simulink model "ALL_JP360_DBW_V6_5_1103"  (R2022a)
settings: Solver=FixedStepAuto  StartTime=0.0  StopTime=inf  FixedStep=0.01  RelTol=1e-3  EnableMultiTasking=on
model workspace (MAT data in the model file):
  g = 9.8
undefined symbols (not defined in the file or in its folder): canChannel, delta_v_p, IPM_Line_C0, IPM_Line_C1, IPM_Line_C2, IPM_Line_C3, M, M_p, MRR_ObjDistX, MRR_ObjDistY, MRR_ObjFusionCamID, MRR_ObjFusionSig, MRR_ObjID, MRR_ObjRelVelX, MRR_ObjRelVelY, MRR_ObjType, MRR_ObjUpdFlg, none, obj_vaild, untracktime, V, videoinput
libraries: canfdmsglib x230, canfdlib x76, slpidlib x24, simulink x18, dspstat3 x14, ctrlSharedLib x1, simulink_extras x1, imaqlib x1, realtime_pacer_lib x1, dspvision x1, visionsinks x1
(part 53 of 55)

== system ALL_JP360_DBW_V6_5_1103/ACC_Control/ACC_FUNCTION/Subsystem2/Limit/acceleration_throttle——PID/Out_PID/Subsystem11 ==
  acce : Inport
  Action Port : ActionPort  InitializeStates=reset  PropagateVarSize=During execution
  Constant : Constant  Value=100
  Constant1 : Constant  OutDataTypeStr=single
  Constant2 : Constant  OutDataTypeStr=uint8
  Constant4 : Constant  OutDataTypeStr=uint8
  P1 : Gain  Gain=0.08
  P3 : Gain  Gain=0.12
  P4 : Gain  Gain=130
  PID Controller : slpidlib/PID Controller  Controller=PID  Form=Parallel  TimeDomain=Continuous-time  UseExternalTs=off  SampleTime=-1  IntegratorMethod=Forward Euler  FilterMethod=Forward Euler  ControllerParametersSource=external  P=1  I=1  UseKiTs=off  D=0  N=100  UseFilter=on  TunerSelectOption=Transfer Function Based (PID Tuner App)  InitialConditionSource=internal  InitialConditionForIntegrator=0  InitialConditionForFilter=0  DifferentiatorICPrevScaledInput=0  ExternalReset=none  TrackingMode=off  Kt=1  LimitOutput=off  SatLimitsSource=internal  UpperSaturationLimit=inf  LowerSaturationLimit=-inf  LinearizeAsGain=on  AntiWindupMode=none  Kb=1  POutMin=[]  POutMax=[]  IOutMin=[]  IOutMax=[]  DOutMin=[]  DOutMax=[]  NOutMin=[]  NOutMax=[]  SumOutDataTypeStr=single  SumOutMin=[]  SumOutMax=[]  SaturationOutMin=[]  SaturationOutMax=[]  PParamMin=[]  PParamMax=[]  IParamMin=[]  IParamMax=[]  DParamMin=[]  DParamMax=[]  NParamMin=[]  NParamMax=[]  KbParamMin=[]  KbParamMax=[]  KtParamMin=[]  KtParamMax=[]  KbOutMin=[]  KbOutMax=[]  KtOutMin=[]  KtOutMax=[]  IntegratorOutMin=[]  IntegratorOutMax=[]  FilterOutMin=[]  FilterOutMax=[]  SumI1OutMin=[]  SumI1OutMax=[]  SumI2OutMin=[]  SumI2OutMax=[]  SumI3OutMin=[]  SumI3OutMax=[]  SumI4OutMin=[]  SumI4OutMax=[]  SumDOutMin=[]  SumDOutMax=[]  DifferentiatorOutMin=[]  DifferentiatorOutMax=[]  FilterDiffOutCoefMin=[]  FilterDiffOutCoefMax=[]  ReciprocalOutMin=[]  ReciprocalOutMax=[]  SumDenOutMin=[]  SumDenOutMax=[]  SumNumOutMin=[]  SumNumOutMax=[]  DivideOutMin=[]  DivideOutMax=[]  UdiffTsProdOutMin=[]  UdiffTsProdOutMax=[]  NTsProdOutMin=[]  NTsProdOutMax=[]  UintegralTsProdOutMin=[]  UintegralTsProdOutMax=[]  UngainTsProdOutMin=[]  UngainTsProdOutMax=[]  IntegratorContinuousStateAttributes=''  IntegratorStateMustResolveToSignalObject=off  IntegratorRTWStateStorageClass=Auto  FilterContinuousStateAttributes=''  FilterStateMustResolveToSignalObject=off  FilterRTWStateStorageClass=Auto  ParallelPVariant=ExternalParameters  IdealPVariant=Disabled  IVariant=ExternalParameters  DVariant=ExternalParameters  IntegratorVariant=Continuous  SatVariant=Disabled  AWVariant=Passthrough  PCopyVariant=Disabled  TRVariant=Disabled  FdbkBlocksVariant=Forward  IdealPFdbkVariant=Disabled  SatFdbkVariant=Disabled  DerivativeFilterVariant=ContFilter  NVariant=ExternalParameters  NCopyVariant=Disabled  FilterICVariant=InternalICsFilter  IntegratorICVariant=InternalICs  ExternalResetVariant=Disabled  TRSumVariant=Passthrough  SumFdbkVariant=Disabled  SumVariant=Sum_PID  TsampFilterVariant=InternalTs  TsampNgainVariant=Passthrough  TsampIntegralVariant=Passthrough  ExternalSaturationOutDataTypeStr=Inherit: Same as second input  aMode=0
  Out1 : Outport
  wires:
  PID Controller/1 -> Out1/1  "throttle"
  acce/1 -> PID Controller/1  "err_v"
  P3/1 -> PID Controller/3
  Constant/1 -> PID Controller/5
  Constant4/1 -> P4/1
  Constant2/1 -> P1/1
  Constant1/1 -> P3/1
  P1/1 -> PID Controller/4
  P4/1 -> PID Controller/2

== system ALL_JP360_DBW_V6_5_1103/ACC_Control/ACC_FUNCTION/Subsystem2/Limit/acceleration_throttle——PID/Out_PID/Subsystem12 ==
  acce : Inport
  Action Port : ActionPort  InitializeStates=reset  PropagateVarSize=During execution
  Constant : Constant  Value=100
  Constant1 : Constant  OutDataTypeStr=single
  Constant2 : Constant  OutDataTypeStr=uint8
  Constant4 : Constant  OutDataTypeStr=uint8
  P1 : Gain  Gain=0.08
  P3 : Gain  Gain=0.12
  P4 : Gain  Gain=130
  PID Controller : slpidlib/PID Controller  Controller=PID  Form=Parallel  TimeDomain=Continuous-time  UseExternalTs=off  SampleTime=-1  IntegratorMethod=Forward Euler  FilterMethod=Forward Euler  ControllerParametersSource=external  P=1  I=1  UseKiTs=off  D=0  N=100  UseFilter=on  TunerSelectOption=Transfer Function Based (PID Tuner App)  InitialConditionSource=internal  InitialConditionForIntegrator=0  InitialConditionForFilter=0  DifferentiatorICPrevScaledInput=0  ExternalReset=none  TrackingMode=off  Kt=1  LimitOutput=off  SatLimitsSource=internal  UpperSaturationLimit=inf  LowerSaturationLimit=-inf  LinearizeAsGain=on  AntiWindupMode=none  Kb=1  POutMin=[]  POutMax=[]  IOutMin=[]  IOutMax=[]  DOutMin=[]  DOutMax=[]  NOutMin=[]  NOutMax=[]  SumOutDataTypeStr=single  SumOutMin=[]  SumOutMax=[]  SaturationOutMin=[]  SaturationOutMax=[]  PParamMin=[]  PParamMax=[]  IParamMin=[]  IParamMax=[]  DParamMin=[]  DParamMax=[]  NParamMin=[]  NParamMax=[]  KbParamMin=[]  KbParamMax=[]  KtParamMin=[]  KtParamMax=[]  KbOutMin=[]  KbOutMax=[]  KtOutMin=[]  KtOutMax=[]  IntegratorOutMin=[]  IntegratorOutMax=[]  FilterOutMin=[]  FilterOutMax=[]  SumI1OutMin=[]  SumI1OutMax=[]  SumI2OutMin=[]  SumI2OutMax=[]  SumI3OutMin=[]  SumI3OutMax=[]  SumI4OutMin=[]  SumI4OutMax=[]  SumDOutMin=[]  SumDOutMax=[]  DifferentiatorOutMin=[]  DifferentiatorOutMax=[]  FilterDiffOutCoefMin=[]  FilterDiffOutCoefMax=[]  ReciprocalOutMin=[]  ReciprocalOutMax=[]  SumDenOutMin=[]  SumDenOutMax=[]  SumNumOutMin=[]  SumNumOutMax=[]  DivideOutMin=[]  DivideOutMax=[]  UdiffTsProdOutMin=[]  UdiffTsProdOutMax=[]  NTsProdOutMin=[]  NTsProdOutMax=[]  UintegralTsProdOutMin=[]  UintegralTsProdOutMax=[]  UngainTsProdOutMin=[]  UngainTsProdOutMax=[]  IntegratorContinuousStateAttributes=''  IntegratorStateMustResolveToSignalObject=off  IntegratorRTWStateStorageClass=Auto  FilterContinuousStateAttributes=''  FilterStateMustResolveToSignalObject=off  FilterRTWStateStorageClass=Auto  ParallelPVariant=ExternalParameters  IdealPVariant=Disabled  IVariant=ExternalParameters  DVariant=ExternalParameters  IntegratorVariant=Continuous  SatVariant=Disabled  AWVariant=Passthrough  PCopyVariant=Disabled  TRVariant=Disabled  FdbkBlocksVariant=Forward  IdealPFdbkVariant=Disabled  SatFdbkVariant=Disabled  DerivativeFilterVariant=ContFilter  NVariant=ExternalParameters  NCopyVariant=Disabled  FilterICVariant=InternalICsFilter  IntegratorICVariant=InternalICs  ExternalResetVariant=Disabled  TRSumVariant=Passthrough  SumFdbkVariant=Disabled  SumVariant=Sum_PID  TsampFilterVariant=InternalTs  TsampNgainVariant=Passthrough  TsampIntegralVariant=Passthrough  ExternalSaturationOutDataTypeStr=Inherit: Same as second input  aMode=0
  Out1 : Outport
  wires:
  P4/1 -> PID Controller/2
  P1/1 -> PID Controller/4
  Constant1/1 -> P3/1
  Constant2/1 -> P1/1
  Constant4/1 -> P4/1
  Constant/1 -> PID Controller/5
  P3/1 -> PID Controller/3
  acce/1 -> PID Controller/1  "err_v"
  PID Controller/1 -> Out1/1  "throttle"

== system ALL_JP360_DBW_V6_5_1103/ACC_Control/ACC_FUNCTION/Subsystem2/Limit/acceleration_throttle——PID/Out_PID/Subsystem13 ==
  Action Port : ActionPort  InitializeStates=reset  PropagateVarSize=During execution
  Constant3 : Constant  Value=25  OutDataTypeStr=uint8
  Data Type Conversion : DataTypeConversion  OutDataTypeStr=single  SaturateOnIntegerOverflow=off  RndMeth=Floor
  Out1 : Outport
  wires:
  Data Type Conversion/1 -> Out1/1
  Constant3/1 -> Data Type Conversion/1  "throttle"

== system ALL_JP360_DBW_V6_5_1103/ACC_Control/ACC_FUNCTION/Subsystem2/Limit/acceleration_throttle——PID/Out_PID/Subsystem2 ==
  Action Port : ActionPort  InitializeStates=reset  PropagateVarSize=During execution
  Constant1 : Constant  Value=0  OutDataTypeStr=single
  Constant3 : Constant  Value=25  OutDataTypeStr=uint8
  Data Type Conversion : DataTypeConversion  OutDataTypeStr=single  SaturateOnIntegerOverflow=off  RndMeth=Floor
  Out1 : Outport
  Out2 : Outport  Port=2
  wires:
  Constant1/1 -> Out2/1  "throttle"
  Constant3/1 -> Data Type Conversion/1  "throttle"
  Data Type Conversion/1 -> Out1/1

== system ALL_JP360_DBW_V6_5_1103/ACC_Control/ACC_FUNCTION/Subsystem2/Limit/acceleration_throttle——PID/Out_PID/up81 ==
  acce : Inport
  Action Port : ActionPort  InitializeStates=reset  PropagateVarSize=During execution
  Constant : Constant  Value=100  OutDataTypeStr=int8
  Constant1 : Constant  OutDataTypeStr=uint16
  Constant2 : Constant  OutDataTypeStr=uint16
  Constant3 : Constant  Value=81  OutDataTypeStr=single
  Constant4 : Constant  OutDataTypeStr=uint8
  P1 : Gain  Gain=0
  P3 : Gain  Gain=6
  P4 : Gain  Gain=145
  PID Controller : slpidlib/PID Controller  Controller=PID  Form=Parallel  TimeDomain=Continuous-time  UseExternalTs=off  SampleTime=-1  IntegratorMethod=Forward Euler  FilterMethod=Forward Euler  ControllerParametersSource=external  P=1  I=1  UseKiTs=off  D=0  N=100  UseFilter=on  TunerSelectOption=Transfer Function Based (PID Tuner App)  InitialConditionSource=internal  InitialConditionForIntegrator=0  InitialConditionForFilter=0  DifferentiatorICPrevScaledInput=0  ExternalReset=none  TrackingMode=off  Kt=1  LimitOutput=off  SatLimitsSource=internal  UpperSaturationLimit=inf  LowerSaturationLimit=-inf  LinearizeAsGain=on  AntiWindupMode=none  Kb=1  POutMin=[]  POutMax=[]  IOutMin=[]  IOutMax=[]  DOutMin=[]  DOutMax=[]  NOutMin=[]  NOutMax=[]  SumOutDataTypeStr=single  SumOutMin=[]  SumOutMax=[]  SaturationOutMin=[]  SaturationOutMax=[]  PParamMin=[]  PParamMax=[]  IParamMin=[]  IParamMax=[]  DParamMin=[]  DParamMax=[]  NParamMin=[]  NParamMax=[]  KbParamMin=[]  KbParamMax=[]  KtParamMin=[]  KtParamMax=[]  KbOutMin=[]  KbOutMax=[]  KtOutMin=[]  KtOutMax=[]  IntegratorOutMin=[]  IntegratorOutMax=[]  FilterOutMin=[]  FilterOutMax=[]  SumI1OutMin=[]  SumI1OutMax=[]  SumI2OutMin=[]  SumI2OutMax=[]  SumI3OutMin=[]  SumI3OutMax=[]  SumI4OutMin=[]  SumI4OutMax=[]  SumDOutMin=[]  SumDOutMax=[]  DifferentiatorOutMin=[]  DifferentiatorOutMax=[]  FilterDiffOutCoefMin=[]  FilterDiffOutCoefMax=[]  ReciprocalOutMin=[]  ReciprocalOutMax=[]  SumDenOutMin=[]  SumDenOutMax=[]  SumNumOutMin=[]  SumNumOutMax=[]  DivideOutMin=[]  DivideOutMax=[]  UdiffTsProdOutMin=[]  UdiffTsProdOutMax=[]  NTsProdOutMin=[]  NTsProdOutMax=[]  UintegralTsProdOutMin=[]  UintegralTsProdOutMax=[]  UngainTsProdOutMin=[]  UngainTsProdOutMax=[]  IntegratorContinuousStateAttributes=''  IntegratorStateMustResolveToSignalObject=off  IntegratorRTWStateStorageClass=Auto  FilterContinuousStateAttributes=''  FilterStateMustResolveToSignalObject=off  FilterRTWStateStorageClass=Auto  ParallelPVariant=ExternalParameters  IdealPVariant=Disabled  IVariant=ExternalParameters  DVariant=ExternalParameters  IntegratorVariant=Continuous  SatVariant=Disabled  AWVariant=Passthrough  PCopyVariant=Disabled  TRVariant=Disabled  FdbkBlocksVariant=Forward  IdealPFdbkVariant=Disabled  SatFdbkVariant=Disabled  DerivativeFilterVariant=ContFilter  NVariant=ExternalParameters  NCopyVariant=Disabled  FilterICVariant=InternalICsFilter  IntegratorICVariant=InternalICs  ExternalResetVariant=Disabled  TRSumVariant=Passthrough  SumFdbkVariant=Disabled  SumVariant=Sum_PID  TsampFilterVariant=InternalTs  TsampNgainVariant=Passthrough  TsampIntegralVariant=Passthrough  ExternalSaturationOutDataTypeStr=Inherit: Same as second input  aMode=0
  Out1 : Outport
  Out2 : Outport  Port=2
  wires:
  Constant3/1 -> Out2/1  "throttle"
  P4/1 -> PID Controller/2
  P1/1 -> PID Controller/4
  Constant1/1 -> P3/1
  Constant2/1 -> P1/1
  Constant4/1 -> P4/1
  Constant/1 -> PID Controller/5
  P3/1 -> PID Controller/3
  acce/1 -> PID Controller/1  "err_v"
  PID Controller/1 -> Out1/1  "throttle"

== system ALL_JP360_DBW_V6_5_1103/ACC_Control/ACC_FUNCTION/Subsystem2/Limit/acceleration_throttle——PID/Subsystem2/30-50 ==
  acce : Inport
  Action Port : ActionPort  InitializeStates=reset  PropagateVarSize=During execution
  Constant : Constant  Value=100
  Constant1 : Constant  OutDataTypeStr=single
  Constant2 : Constant  OutDataTypeStr=uint8
  Constant3 : Constant  Value=100  OutDataTypeStr=single
  Constant4 : Constant  OutDataTypeStr=uint8
  P1 : Gain  Gain=0
  P3 : Gain  Gain=3
  P4 : Gain  Gain=110
  PID Controller : slpidlib/PID Controller  Controller=PID  Form=Parallel  TimeDomain=Continuous-time  UseExternalTs=off  SampleTime=-1  IntegratorMethod=Forward Euler  FilterMethod=Forward Euler  ControllerParametersSource=external  P=1  I=1  UseKiTs=off  D=0  N=100  UseFilter=on  TunerSelectOption=Transfer Function Based (PID Tuner App)  InitialConditionSource=internal  InitialConditionForIntegrator=0  InitialConditionForFilter=0  DifferentiatorICPrevScaledInput=0  ExternalReset=none  TrackingMode=off  Kt=1  LimitOutput=off  SatLimitsSource=internal  UpperSaturationLimit=inf  LowerSaturationLimit=-inf  LinearizeAsGain=on  AntiWindupMode=none  Kb=1  POutMin=[]  POutMax=[]  IOutMin=[]  IOutMax=[]  DOutMin=[]  DOutMax=[]  NOutMin=[]  NOutMax=[]  SumOutDataTypeStr=single  SumOutMin=[]  SumOutMax=[]  SaturationOutMin=[]  SaturationOutMax=[]  PParamMin=[]  PParamMax=[]  IParamMin=[]  IParamMax=[]  DParamMin=[]  DParamMax=[]  NParamMin=[]  NParamMax=[]  KbParamMin=[]  KbParamMax=[]  KtParamMin=[]  KtParamMax=[]  KbOutMin=[]  KbOutMax=[]  KtOutMin=[]  KtOutMax=[]  IntegratorOutMin=[]  IntegratorOutMax=[]  FilterOutMin=[]  FilterOutMax=[]  SumI1OutMin=[]  SumI1OutMax=[]  SumI2OutMin=[]  SumI2OutMax=[]  SumI3OutMin=[]  SumI3OutMax=[]  SumI4OutMin=[]  SumI4OutMax=[]  SumDOutMin=[]  SumDOutMax=[]  DifferentiatorOutMin=[]  DifferentiatorOutMax=[]  FilterDiffOutCoefMin=[]  FilterDiffOutCoefMax=[]  ReciprocalOutMin=[]  ReciprocalOutMax=[]  SumDenOutMin=[]  SumDenOutMax=[]  SumNumOutMin=[]  SumNumOutMax=[]  DivideOutMin=[]  DivideOutMax=[]  UdiffTsProdOutMin=[]  UdiffTsProdOutMax=[]  NTsProdOutMin=[]  NTsProdOutMax=[]  UintegralTsProdOutMin=[]  UintegralTsProdOutMax=[]  UngainTsProdOutMin=[]  UngainTsProdOutMax=[]  IntegratorContinuousStateAttributes=''  IntegratorStateMustResolveToSignalObject=off  IntegratorRTWStateStorageClass=Auto  FilterContinuousStateAttributes=''  FilterStateMustResolveToSignalObject=off  FilterRTWStateStorageClass=Auto  ParallelPVariant=ExternalParameters  IdealPVariant=Disabled  IVariant=ExternalParameters  DVariant=ExternalParameters  IntegratorVariant=Continuous  SatVariant=Disabled  AWVariant=Passthrough  PCopyVariant=Disabled  TRVariant=Disabled  FdbkBlocksVariant=Forward  IdealPFdbkVariant=Disabled  SatFdbkVariant=Disabled  DerivativeFilterVariant=ContFilter  NVariant=ExternalParameters  NCopyVariant=Disabled  FilterICVariant=InternalICsFilter  IntegratorICVariant=InternalICs  ExternalResetVariant=Disabled  TRSumVariant=Passthrough  SumFdbkVariant=Disabled  SumVariant=Sum_PID  TsampFilterVariant=InternalTs  TsampNgainVariant=Passthrough  TsampIntegralVariant=Passthrough  ExternalSaturationOutDataTypeStr=Inherit: Same as second input  aMode=0
  Out1 : Outport
  Out2 : Outport  Port=2
  wires:
  Constant3/1 -> Out2/1
  P4/1 -> PID Controller/2
  P1/1 -> PID Controller/4
  Constant1/1 -> P3/1
  Constant2/1 -> P1/1
  Constant4/1 -> P4/1
  Constant/1 -> PID Controller/5
  P3/1 -> PID Controller/3
  acce/1 -> PID Controller/1  "err_v"
  PID Controller/1 -> Out1/1  "throttle"

== system ALL_JP360_DBW_V6_5_1103/ACC_Control/ACC_FUNCTION/Subsystem2/Limit/acceleration_throttle——PID/Subsystem2/51-80 ==
  acce : Inport
  Action Port : ActionPort  InitializeStates=reset  PropagateVarSize=During execution
  Constant : Constant  Value=100
  Constant1 : Constant  OutDataTypeStr=single
  Constant2 : Constant  OutDataTypeStr=uint8
  Constant3 : Constant  Value=200  OutDataTypeStr=single
  Constant4 : Constant  OutDataTypeStr=uint8
  P1 : Gain  Gain=0
  P3 : Gain  Gain=5
  P4 : Gain  Gain=135
  PID Controller : slpidlib/PID Controller  Controller=PID  Form=Parallel  TimeDomain=Continuous-time  UseExternalTs=off  SampleTime=-1  IntegratorMethod=Forward Euler  FilterMethod=Forward Euler  ControllerParametersSource=external  P=1  I=1  UseKiTs=off  D=0  N=100  UseFilter=on  TunerSelectOption=Transfer Function Based (PID Tuner App)  InitialConditionSource=internal  InitialConditionForIntegrator=0  InitialConditionForFilter=0  DifferentiatorICPrevScaledInput=0  ExternalReset=none  TrackingMode=off  Kt=1  LimitOutput=off  SatLimitsSource=internal  UpperSaturationLimit=inf  LowerSaturationLimit=-inf  LinearizeAsGain=on  AntiWindupMode=none  Kb=1  POutMin=[]  POutMax=[]  IOutMin=[]  IOutMax=[]  DOutMin=[]  DOutMax=[]  NOutMin=[]  NOutMax=[]  SumOutDataTypeStr=single  SumOutMin=[]  SumOutMax=[]  SaturationOutMin=[]  SaturationOutMax=[]  PParamMin=[]  PParamMax=[]  IParamMin=[]  IParamMax=[]  DParamMin=[]  DParamMax=[]  NParamMin=[]  NParamMax=[]  KbParamMin=[]  KbParamMax=[]  KtParamMin=[]  KtParamMax=[]  KbOutMin=[]  KbOutMax=[]  KtOutMin=[]  KtOutMax=[]  IntegratorOutMin=[]  IntegratorOutMax=[]  FilterOutMin=[]  FilterOutMax=[]  SumI1OutMin=[]  SumI1OutMax=[]  SumI2OutMin=[]  SumI2OutMax=[]  SumI3OutMin=[]  SumI3OutMax=[]  SumI4OutMin=[]  SumI4OutMax=[]  SumDOutMin=[]  SumDOutMax=[]  DifferentiatorOutMin=[]  DifferentiatorOutMax=[]  FilterDiffOutCoefMin=[]  FilterDiffOutCoefMax=[]  ReciprocalOutMin=[]  ReciprocalOutMax=[]  SumDenOutMin=[]  SumDenOutMax=[]  SumNumOutMin=[]  SumNumOutMax=[]  DivideOutMin=[]  DivideOutMax=[]  UdiffTsProdOutMin=[]  UdiffTsProdOutMax=[]  NTsProdOutMin=[]  NTsProdOutMax=[]  UintegralTsProdOutMin=[]  UintegralTsProdOutMax=[]  UngainTsProdOutMin=[]  UngainTsProdOutMax=[]  IntegratorContinuousStateAttributes=''  IntegratorStateMustResolveToSignalObject=off  IntegratorRTWStateStorageClass=Auto  FilterContinuousStateAttributes=''  FilterStateMustResolveToSignalObject=off  FilterRTWStateStorageClass=Auto  ParallelPVariant=ExternalParameters  IdealPVariant=Disabled  IVariant=ExternalParameters  DVariant=ExternalParameters  IntegratorVariant=Continuous  SatVariant=Disabled  AWVariant=Passthrough  PCopyVariant=Disabled  TRVariant=Disabled  FdbkBlocksVariant=Forward  IdealPFdbkVariant=Disabled  SatFdbkVariant=Disabled  DerivativeFilterVariant=ContFilter  NVariant=ExternalParameters  NCopyVariant=Disabled  FilterICVariant=InternalICsFilter  IntegratorICVariant=InternalICs  ExternalResetVariant=Disabled  TRSumVariant=Passthrough  SumFdbkVariant=Disabled  SumVariant=Sum_PID  TsampFilterVariant=InternalTs  TsampNgainVariant=Passthrough  TsampIntegralVariant=Passthrough  ExternalSaturationOutDataTypeStr=Inherit: Same as second input  aMode=0
  Out1 : Outport
  Out2 : Outport  Port=2
  wires:
  Constant3/1 -> Out2/1
  PID Controller/1 -> Out1/1  "throttle"
  acce/1 -> PID Controller/1  "err_v"
  P3/1 -> PID Controller/3
  Constant/1 -> PID Controller/5
  Constant4/1 -> P4/1
  Constant2/1 -> P1/1
  Constant1/1 -> P3/1
  P1/1 -> PID Controller/4
  P4/1 -> PID Controller/2

== system ALL_JP360_DBW_V6_5_1103/ACC_Control/ACC_FUNCTION/Subsystem2/Limit/acceleration_throttle——PID/Subsystem2/up81 ==
  acce : Inport
  Action Port : ActionPort  InitializeStates=reset  PropagateVarSize=During execution
  Constant : Constant  Value=100  OutDataTypeStr=int8
  Constant1 : Constant  OutDataTypeStr=uint16
  Constant2 : Constant  OutDataTypeStr=uint16
  Constant3 : Constant  Value=300  OutDataTypeStr=single
  Constant4 : Constant  OutDataTypeStr=uint8
  P1 : Gain  Gain=0
  P3 : Gain  Gain=5.5
  P4 : Gain  Gain=130
  PID Controller : slpidlib/PID Controller  Controller=PID  Form=Parallel  TimeDomain=Continuous-time  UseExternalTs=off  SampleTime=-1  IntegratorMethod=Forward Euler  FilterMethod=Forward Euler  ControllerParametersSource=external  P=1  I=1  UseKiTs=off  D=0  N=100  UseFilter=on  TunerSelectOption=Transfer Function Based (PID Tuner App)  InitialConditionSource=internal  InitialConditionForIntegrator=0  InitialConditionForFilter=0  DifferentiatorICPrevScaledInput=0  ExternalReset=none  TrackingMode=off  Kt=1  LimitOutput=off  SatLimitsSource=internal  UpperSaturationLimit=inf  LowerSaturationLimit=-inf  LinearizeAsGain=on  AntiWindupMode=none  Kb=1  POutMin=[]  POutMax=[]  IOutMin=[]  IOutMax=[]  DOutMin=[]  DOutMax=[]  NOutMin=[]  NOutMax=[]  SumOutDataTypeStr=single  SumOutMin=[]  SumOutMax=[]  SaturationOutMin=[]  SaturationOutMax=[]  PParamMin=[]  PParamMax=[]  IParamMin=[]  IParamMax=[]  DParamMin=[]  DParamMax=[]  NParamMin=[]  NParamMax=[]  KbParamMin=[]  KbParamMax=[]  KtParamMin=[]  KtParamMax=[]  KbOutMin=[]  KbOutMax=[]  KtOutMin=[]  KtOutMax=[]  IntegratorOutMin=[]  IntegratorOutMax=[]  FilterOutMin=[]  FilterOutMax=[]  SumI1OutMin=[]  SumI1OutMax=[]  SumI2OutMin=[]  SumI2OutMax=[]  SumI3OutMin=[]  SumI3OutMax=[]  SumI4OutMin=[]  SumI4OutMax=[]  SumDOutMin=[]  SumDOutMax=[]  DifferentiatorOutMin=[]  DifferentiatorOutMax=[]  FilterDiffOutCoefMin=[]  FilterDiffOutCoefMax=[]  ReciprocalOutMin=[]  ReciprocalOutMax=[]  SumDenOutMin=[]  SumDenOutMax=[]  SumNumOutMin=[]  SumNumOutMax=[]  DivideOutMin=[]  DivideOutMax=[]  UdiffTsProdOutMin=[]  UdiffTsProdOutMax=[]  NTsProdOutMin=[]  NTsProdOutMax=[]  UintegralTsProdOutMin=[]  UintegralTsProdOutMax=[]  UngainTsProdOutMin=[]  UngainTsProdOutMax=[]  IntegratorContinuousStateAttributes=''  IntegratorStateMustResolveToSignalObject=off  IntegratorRTWStateStorageClass=Auto  FilterContinuousStateAttributes=''  FilterStateMustResolveToSignalObject=off  FilterRTWStateStorageClass=Auto  ParallelPVariant=ExternalParameters  IdealPVariant=Disabled  IVariant=ExternalParameters  DVariant=ExternalParameters  IntegratorVariant=Continuous  SatVariant=Disabled  AWVariant=Passthrough  PCopyVariant=Disabled  TRVariant=Disabled  FdbkBlocksVariant=Forward  IdealPFdbkVariant=Disabled  SatFdbkVariant=Disabled  DerivativeFilterVariant=ContFilter  NVariant=ExternalParameters  NCopyVariant=Disabled  FilterICVariant=InternalICsFilter  IntegratorICVariant=InternalICs  ExternalResetVariant=Disabled  TRSumVariant=Passthrough  SumFdbkVariant=Disabled  SumVariant=Sum_PID  TsampFilterVariant=InternalTs  TsampNgainVariant=Passthrough  TsampIntegralVariant=Passthrough  ExternalSaturationOutDataTypeStr=Inherit: Same as second input  aMode=0
  Out1 : Outport
  Out2 : Outport  Port=2
  wires:
  Constant3/1 -> Out2/1
  P4/1 -> PID Controller/2
  P1/1 -> PID Controller/4
  Constant1/1 -> P3/1
  Constant2/1 -> P1/1
  Constant4/1 -> P4/1
  Constant/1 -> PID Controller/5
  P3/1 -> PID Controller/3
  acce/1 -> PID Controller/1  "err_v"
  PID Controller/1 -> Out1/1  "throttle"

== system ALL_JP360_DBW_V6_5_1103/ACC_Control/ACC_FUNCTION/Subsystem2/ACC_model/TIS1 ACC action/Subsystem1/mode change/cc ==
  throttle_in : Inport
  brake_in : Inport  Port=2
  Action Port : ActionPort  InitializeStates=reset  PropagateVarSize=During execution  ActionPortLabel=if(u1 > 0)
  Constant : Constant  Value=2  OutDataTypeStr=single
  acceleration [a] : Outport  InitialOutput=[0]
  deceleration [-a] : Outport  Port=2  InitialOutput=[150]
  ACC_MODE : Outport  Port=3  InitialOutput=[150]
  wires:
  brake_in/1 -> deceleration [-a]/1
  throttle_in/1 -> acceleration [a]/1
  Constant/1 -> ACC_MODE/1

== system ALL_JP360_DBW_V6_5_1103/ACC_Control/ACC_FUNCTION/Subsystem2/ACC_model/TIS1 ACC action/Subsystem1/mode change/cc and close and follow ==
  a_zero : Inport
  v_obj : Inport  Port=2
  v_ego : Inport  Port=3
  cc_throttle : Inport  Port=4
  cc_brake : Inport  Port=5
  delta_d_ego : Inport  Port=6
  dx : Inport  Port=7
  Action Port : ActionPort  InitializeStates=reset  PropagateVarSize=During execution  ActionPortLabel=else
  Demux : Demux  Outputs=3
  Merge : Merge
  Mux : Mux  Inputs=3
  Mux2 : Mux  Inputs=3
  cc and close : Subsystem  TreatAsAtomicUnit=on
  follow : Subsystem  TreatAsAtomicUnit=on
  if : If
  acceleration [a] : Outport
  deceleration [-a] : Outport  Port=2
  ACC_MODE : Outport  Port=3
  standstill_req : Outport  Port=4  InitialOutput=[150]
  wires:
  follow/1(acceleration [a]) -> Mux2/1
  if/1 -> cc and close/Action
  Demux/1 -> acceleration [a]/1
  cc and close/2(deceleration [-a]) -> Mux/2
  follow/2(deceleration [-a]) -> Mux2/2
  cc and close/1(acceleration [a]) -> Mux/1
  Merge/1 -> Demux/1
  if/2 -> follow/Action
  Mux/1 -> Merge/1
  Demux/2 -> deceleration [-a]/1
  Mux2/1 -> Merge/2
  v_obj/1 -> cc and close/1(v_obj)
  v_ego/1 -> cc and close/2(v_ego)
  a_zero/1 -> follow/1(brake), if/1
  cc_throttle/1 -> cc and close/3(cc_throttle)
  cc_brake/1 -> cc and close/4(cc_brake)
  delta_d_ego/1 -> cc and close/5(delta_d_ego)
  follow/3(ACC_MODE) -> Mux2/3
  cc and close/3(ACC_MODE) -> Mux/3
  Demux/3 -> ACC_MODE/1
  cc and close/4(standstill_req) -> standstill_req/1
  dx/1 -> cc and close/6(dx)

== system ALL_JP360_DBW_V6_5_1103/ACC_Control/ACC_FUNCTION/Subsystem2/ACC_model/TIS1 ACC action/Subsystem1/mode change/cc and close and follow/cc and close ==
  v_obj : Inport
  v_ego : Inport  Port=2
  cc_throttle : Inport  Port=3
  cc_brake : Inport  Port=4
  delta_d_ego : Inport  Port=5
  dx : Inport  Port=6
  Action Port : ActionPort  InitializeStates=reset  PropagateVarSize=During execution  ActionPortLabel=if(u1 > 0)
  Demux : Demux  Outputs=3
  Merge : Merge
  Mux : Mux  Inputs=3
  Mux2 : Mux  Inputs=3
  Sum : Sum  Inputs=|+-
  cc : Subsystem  TreatAsAtomicUnit=on
  if : If
  move close : Subsystem  TreatAsAtomicUnit=on
  acceleration [a] : Outport  OutDataTypeStr=single  InitialOutput=[0]
  deceleration [-a] : Outport  Port=2  OutDataTypeStr=single  InitialOutput=[150]
  ACC_MODE : Outport  Port=3  OutDataTypeStr=single  InitialOutput=[150]
  standstill_req : Outport  Port=4  InitialOutput=[150]
  wires:
  move close/1(acceleration [a]) -> Mux2/1
  Mux2/1 -> Merge/2
  Mux/1 -> Merge/1
  Merge/1 -> Demux/1
  cc/2(deceleration [-a]) -> Mux/2
  if/2 -> move close/Action
  if/1 -> cc/Action
  move close/2(decleration [-a]) -> Mux2/2
  Demux/2 -> deceleration [-a]/1
  Demux/1 -> acceleration [a]/1
  v_obj/1 -> move close/3(v_obj), Sum/1
  v_ego/1 -> move close/4(v_ego), Sum/2
  Sum/1 -> move close/2(delta_v), if/1
  cc_throttle/1 -> cc/1(cc_throttle), move close/5(cc_throttle)
  cc_brake/1 -> move close/6(cc_brake), cc/2(cc_brake)
  delta_d_ego/1 -> move close/1(delta_d_ego)
  cc/3(ACC_MODE) -> Mux/3
  move close/3(ACC_MODE) -> Mux2/3
  Demux/3 -> ACC_MODE/1
  cc/1(acceleration [a]) -> Mux/1
  move close/4(standstill_req) -> standstill_req/1
  dx/1 -> move close/7(dx)

== system ALL_JP360_DBW_V6_5_1103/ACC_Control/ACC_FUNCTION/Subsystem2/ACC_model/TIS1 ACC action/Subsystem1/mode change/cc and close and follow/follow ==
  brake : Inport
  Action Port : ActionPort  InitializeStates=reset  PropagateVarSize=During execution  ActionPortLabel=else
  Constant : Constant  Value=0  OutDataTypeStr=single
  Constant1 : Constant  Value=4  OutDataTypeStr=single
  Saturation : Saturate  UpperLimit=0  LowerLimit=-8
  acceleration [a] : Outport  InitialOutput=[0]
  deceleration [-a] : Outport  Port=2  InitialOutput=[150]
  ACC_MODE : Outport  Port=3  InitialOutput=[0]
  wires:
  Constant/1 -> acceleration [a]/1
  brake/1 -> Saturation/1
  Constant1/1 -> ACC_MODE/1
  Saturation/1 -> deceleration [-a]/1

== system ALL_JP360_DBW_V6_5_1103/ACC_Control/ACC_FUNCTION/Subsystem2/ACC_model/TIS1 ACC action/Subsystem1/mode change/cc and close and follow/cc and close/cc ==
  cc_throttle : Inport
  cc_brake : Inport  Port=2
  Action Port : ActionPort  InitializeStates=reset  PropagateVarSize=During execution  ActionPortLabel=if(u1 > 0)
  Constant : Constant  Value=2  OutDataTypeStr=single
  acceleration [a] : Outport  InitialOutput=[0]
  deceleration [-a] : Outport  Port=2  InitialOutput=[150]
  ACC_MODE : Outport  Port=3  InitialOutput=[150]
  wires:
  cc_throttle/1 -> acceleration [a]/1
  cc_brake/1 -> deceleration [-a]/1
  Constant/1 -> ACC_MODE/1

== system ALL_JP360_DBW_V6_5_1103/ACC_Control/ACC_FUNCTION/Subsystem2/ACC_model/TIS1 ACC action/Subsystem1/mode change/cc and close and follow/cc and close/move close ==
  note: 跟停前车时，若在跟进模式下，目标车静止<10kph，且自车车速＜2kph，发出standstill请求
  delta_d_ego : Inport
  delta_v : Inport  Port=2
  v_obj : Inport  Port=3
  v_ego : Inport  Port=4
  cc_throttle : Inport  Port=5
  cc_brake : Inport  Port=6
  dx : Inport  Port=7
  Action Port : ActionPort  InitializeStates=reset  PropagateVarSize=During execution  ActionPortLabel=else
  AND : Logic  Inputs=3  IconShape=distinctive  AllPortsSameDT=off  OutDataTypeStr=boolean
  Abs2 : Abs  Commented=on  SaturateOnIntegerOverflow=off
  Abs3 : Abs  Commented=on  SaturateOnIntegerOverflow=off
  Constant1 : Constant  Value=3  OutDataTypeStr=single
  Constant2 : Constant  Value=10
  Constant4 : Constant  Value=5/3.6
  Constant5 : Constant  Value=2/3.6
  Divide1 : Product  Inputs=*/
  Gain2 : Gain  Gain=-2
  MATLAB Function : MATLAB Function  TreatAsAtomicUnit=on
  MATLAB Function1 : MATLAB Function  TreatAsAtomicUnit=on
  MATLAB Function2 : MATLAB Function  Commented=on  TreatAsAtomicUnit=on
  Math Function2 : Math  Operator=square
  Relational Operator : RelationalOperator  Operator=<=  OutDataTypeStr=boolean  RndMeth=Simplest  InputSameDT=off
  Relational Operator1 : RelationalOperator  Operator=<=  OutDataTypeStr=boolean  RndMeth=Simplest  InputSameDT=off
  Relational Operator2 : RelationalOperator  Operator=<=  OutDataTypeStr=boolean  RndMeth=Simplest  InputSameDT=off
  Saturation : Saturate  UpperLimit=0  LowerLimit=-8
  Scope : Scope  NumInputPorts=3
  Switch : Switch  Criteria=u2 > Threshold  SaturateOnIntegerOverflow=off  InputSameDT=off
  Switch1 : Switch  Commented=on  Criteria=u2 > Threshold  Threshold=1  SaturateOnIntegerOverflow=off  InputSameDT=off
  a_dem : Constant  Value=0.5  OutDataTypeStr=single
  stand_req demand1 : Constant  OutDataTypeStr=boolean
  stand_req no demand : Constant  Value=0  OutDataTypeStr=boolean
  acceleration [a] : Outport  InitialOutput=[0]
  decleration [-a] : Outport  Port=2  InitialOutput=[150]
  ACC_MODE : Outport  Port=3  InitialOutput=[150]
  standstill_req : Outport  Port=4  InitialOutput=[150]
  wires:
  Abs3/1 -> Switch1/3
  ? -> Abs2/1
  ? -> Abs3/1
  ? -> Switch1/1
  Abs2/1 -> Switch1/2
  Gain2/1 -> Divide1/2
  Math Function2/1 -> Divide1/1
  MATLAB Function/1(y) -> Gain2/1
  Constant1/1 -> ACC_MODE/1
  Saturation/1 -> Scope/2, decleration [-a]/1
  AND/1 -> Switch/2
  stand_req no demand/1 -> Switch/3
  Switch/1 -> standstill_req/1
  Relational Operator/1 -> AND/1
  Relational Operator1/1 -> AND/2
  Constant4/1 -> Relational Operator1/2
  Constant5/1 -> Relational Operator/2
  stand_req demand1/1 -> Switch/1
  v_ego/1 -> Relational Operator/1
  v_obj/1 -> Relational Operator1/1
  delta_d_ego/1 -> [delta_d_ego]
  delta_v/1 -> [delta_v]
  [delta_v] -> Math Function2/1
  [delta_d_ego] -> MATLAB Function/1(delta_d)
  [delta_v] -> MATLAB Function1/1(delta_v)
  dx/1 -> MATLAB Function1/2(dx)
  a_dem/1 -> MATLAB Function1/3(a_dem)
  Divide1/1 -> Scope/3, MATLAB Function1/4(a_close)
  cc_throttle/1 -> MATLAB Function1/5(cc_throttle)
  cc_brake/1 -> MATLAB Function1/6(cc_brake)
  MATLAB Function1/1(acc) -> Scope/1, acceleration [a]/1
  MATLAB Function1/2(dec) -> Saturation/1
  [delta_d_ego] -> Relational Operator2/1
  Relational Operator2/1 -> AND/3
  Constant2/1 -> Relational Operator2/2

== stateflow chart ALL_JP360_DBW_V6_5_1103/ACC_Control/ACC_FUNCTION/Subsystem2/Limit/acceleration_throttle——PID/Out_PID/Subsystem/Chart ==
  state start
    state init
      t=a;
    state init1
      t=b;
    state init2
      t=c;
    state init3
    start -> (junction 8)
    (default) -> (junction 8)
    (junction 8) -> init [order 1] : [s==1]
    (junction 8) -> init2 [order 3] : [s==3]
    (junction 8) -> init1 [order 2] : [s==2]
    (junction 8) -> init3 [order 4]
  (default) -> start
  data: s input; a input single; b input single; c input single; t output single

== stateflow chart ALL_JP360_DBW_V6_5_1103/ACC_Control/ACC_FUNCTION/acc_stateflow/Chart3 ==
  state OFF
    en:y=0;
    en:ACC_DriveOff=0;
  state ON
    en:ACC_DriveOff=1;
    en:y=y+t;
    du:y=y+t
  (default) -> OFF
  OFF -> ON [order 2] : [EMS_IndicatedDriverOverride==1&&ACC_Status==6]{t=0}
  OFF -> ON [order 1] : [((hasChangedFrom(u1,0)&&three_s==0&&((Obj_Speed>5&&ACC_ObjDetected==1)||ACC_ObjDetected==0||(Obj_Speed<=5&&ACC_ObjDetected==1&&CIPV_ObjDistX>=6)))&&ACC_Status==6)||(((ACC_ObjDetected==1&&Obj_Speed>5))&&three_s==1&&ACC_Status==6)]{t=1}
  ON -> OFF : [(y>=250&&t==1)||(EMS_IndicatedDriverOverride==0&&t==0)]
  data: u1 input boolean; y local; ACC_DriveOff output; ACC_Status input; EMS_IndicatedDriverOverride input; ACC_ObjDetected input; Obj_Speed input; t local; three_s input; CIPV_ObjDistX input

== matlab function ALL_JP360_DBW_V6_5_1103/DCLC1/LQR/err kappa calculate module ==
  data: kr output; vx input; xr input; yr input; thetar input; kappar input; err output
function [kr, err] = fcn(vx,xr, yr,thetar,kappar)
%%%%%%%%%%%%%%%%%%%%%%%%%%%%%%%%1、确定预瞄点%%%%%%%%%%%%%%%%%%%%%%%%%%%%%%%%
%%%基本思路为：先根据最近原则找到车辆当前点与参考轨迹上距离最近的匹配点，获取匹配点的索引
%%%然后在匹配点之后取预瞄点，这里要设置一个预瞄窗口，preview_window
%%%在JMC的AVP项目中，泊车场景的预瞄窗口为parking_preview_window=120，行车的预瞄窗口为driving_preview_window=10，
%%%泊出的预瞄窗口为summon_preview_window=10；
% driving_preview_window=1;
% %summon_preview_window=10;
% %parking_preview_window=120;
% n = length(xr);
% d_min = (vehicle_x-xr(1))^2 + (vehicle_y-yr(1))^2; % 根据距离最近原则计算车辆当前点与参考轨迹上连线距离最近点（匹配点）的距离
% min = 1;
% for i = 1:n % 遍历参考轨迹上的所有的点，i为点的索引值
%     d = (vehicle_x-xr(i))^2 + (vehicle_y-yr(i))^2;
%     if d < d_min
%         d_min = d;
%         min = i;
%     end
% end
% dmin = min;  % 遍历参考轨迹，dmin为车辆当前位置与参考轨迹上距离最近的点（匹配点）在轨迹上的索引，相当于找到了匹配点的索引
% preview_point_index_1 = min + driving_preview_window;
% if preview_point_index_1 < n
%    preview_point_index = preview_point_index_1;  % 参考轨迹上预瞄点的索引值
% else
%    preview_point_index = n ;
% end

%%%%%%%%%%%%%%%%%%%%%%%%%2、计算横向偏差和纵向位置偏差%%%%%%%%%%%%%%%%%%%%%%%%%
%     tor=[cos(thetar);sin(thetar)];   % 计算纵向偏差的转换关系
%     nor=[-sin(thetar);cos(thetar)];  % 计算横向偏差的转换关系
%     d_err=[vehicle_x-xr;vehicle_y-yr]; % d_err代表的是车辆当前坐标与跟踪点的坐标在笛卡尔坐标系下横纵坐标的差值，在C++代码分别用dx dy表示
%     ed=-nor'*d_err;     % ed为在frenet坐标系下车辆当前点与轨迹跟踪点的横向误差；
%     es=tor'*d_err;     % es为在frenet坐标系下车辆当前点与轨迹跟踪点的纵向位置误差；
      ed = yr;
%       es = xr;
    
%%%%%%%%%%%%%%%%%%%%%%3、确定预瞄点的航向，直接取预瞄点的航向%%%%%%%%%%%%%%%%%%%
%     projection_point_thetar=thetar;%apollo
    %projection_point_thetar=thetar(dmin)+kappar(dmin)*es;  % projection_point_thetar车辆投影点的航向角
    
%%%%%%%%%%%%4、计算横向误差变化率、航向误差、航向误差变化率、参考曲率%%%%%%%%%%%%
%     ed_dot=vy*cos(thetar)+vx*sin(thetar);% ed_dot横向误差变化率
    %%%%%%%%%
    ephi = thetar; % ephi航向误差
%     ephi=phi-projection_point_thetar;       % ephi航向误差为车辆当前点的航向与预瞄点的航向差值
    %%%%%%%%%

%     ss_dot=vx*cos(phi-projection_point_thetar)-vy*sin(phi-projection_point_thetar);
%     s_dot=ss_dot/(1-kappar*ed);    % 为预瞄点处的速度
%     ephi_dot=phi_dot-kappar*s_dot; % ephi_dot航向误差变化率
%     ephi_dot=kappar*vx; % ephi_dot航向误差变化率
    kr=kappar;                     % kr参考曲率
    err=[ed;0;ephi;0];
 
%%%%%%%%%%%%%%%%%%%%%%%%%%%5、评价跟踪效果：应该计算当前点与匹配点的横向误差、航向误差%%%%%%%%%%%%%%%%%%%%%%%%%%
% % 1、计算车辆当前点与匹配点在笛卡尔坐标系下的横纵坐标差值d_err_match
% tor_match=[cos(thetar(dmin));sin(thetar(dmin))];   % 计算纵向偏差的转换关系
% nor_match = [-sin(thetar(dmin));cos(thetar(dmin))];  % 计算横向偏差的转换关系
% d_err_match = [vehicle_x-xr(dmin);vehicle_y-yr(dmin)]; % d_err代表的是车辆当前坐标与跟踪点的坐标在笛卡尔坐标系下横纵坐标的差值，在C++代码分别用dx dy表示
% 
% % 2、计算当前点与匹配点的ed_match、es_match、ephi_match
% ed_match = nor_match'*d_err_match;     % ed为在frenet坐标系下车辆当前点与轨迹跟踪点的横向误差；
% es_match = tor_match'*d_err_match;     % es为在frenet坐标系下车辆当前点与轨迹跟踪点的纵向位置误差；
% ephi_match = phi - thetar(dmin);
% err_match = [ed_match;es_match;ephi_match];
% 
% 
%     % ed:横向偏差
%     % ed_dot：横向偏差变化率
%     % ephi：航向偏差
%     % ephi_dot：航向偏差变化率     
end

== matlab function ALL_JP360_DBW_V6_5_1103/DCLC1/LQR/forward_angle1 ==
  data: a input; b input; m input; cf input; cr input; vx input; forward_angle output; k input; kr input; ephi input
function forward_angle = fcn(a,b,m,cf,cr,vx,k,kr,ephi)
   %前馈方法1-------时工(基于曲率补偿的方法)
   forward_angle= -(a+b)*kr;
   
   %前馈方法2-------(glx论文) 如果侧偏刚度为正 forward_angle= -0.95 * ephi
   % forward_angle= 0.95 * ephi;%侧偏刚度为负
   
   %前馈方法3-------(基于拉氏变换和终值定理的前馈控制)，这里侧偏刚度为负值
   % forward_angle=kr*(a+b-b*k(3)+(m*vx*vx/(a+b))*((b/cf)+(a/cr)*k(3)-(a/cr)));
   
   %前馈方法4-------(自适应前馈控制)
%     forward_angle= kr*(m*vx*vx+a*cf-b*cr)/cf;
   
   %前馈方法5-------(基于二自由度模型横摆稳态响应特性的前馈控制)，这里侧偏刚度为负值
   %forward_angle= -(vx*kr/(vx/(a+b))/(1+m/(a+b)/(a+b)*(a/cr-b/cf)*vx*vx));
   
end
%注意：仿真里面侧偏刚度用得是负值，Apollo，JMC里面侧偏刚度用的是正值，但是前馈理论都是基于侧偏刚度为正值来推理的
%故需要对以上策略再添加一个负号

== matlab function ALL_JP360_DBW_V6_5_1103/DCLC1/MATLAB Function ==
  data: ACC_Enable input; u output
function u = fcn(ACC_Enable)

% 0: OFF 
% 1: Passive 
% 2: Stand-By 
% 3: Active-Control 
% 5: Override 
% 6:Standstill 
% 7:Failure

if ACC_Enable == 3
    u = 1;
else
    u = 0;
end

== matlab function ALL_JP360_DBW_V6_5_1103/DCLC1/MATLAB Function1 ==
  data: LKA_Enable input; u output
function u = fcn(LKA_Enable)

% 0: OFF 
% 1: PASSIVE/STANDBY 
% 4: ACTIVE 
% 5: ERROR

if LKA_Enable == 4
    u = 1;
else
    u = 0;
end

== matlab function ALL_JP360_DBW_V6_5_1103/CIPV1/Lane Line Construction1/Embedded MATLAB Function6 ==
  data: R input; SteerWheelAngle input; line_data output; IPM_Line_type input
function line_data = line_count_fun(R, SteerWheelAngle, IPM_Line_type)

if IPM_Line_type==2   %左车道线是道路边缘，所以无左左车道线
    line_data = single([0, 0, 0, 0]);
else
    if R>100
        line_data = single([5.625, 0, 0, 0]);
    else
        if SteerWheelAngle < 0  %turn right
            IPM_Line_C0 = 5.625;
            IPM_Line_C1 = 0;
            IPM_Line_C2 = -(1/(R+5.625));
            line_data = single([IPM_Line_C0, IPM_Line_C1, IPM_Line_C2, 0]);
        else
            IPM_Line_C0 = 5.625;
            IPM_Line_C1 = 0;
            IPM_Line_C2 = 1/(R-5.625);
            line_data = single([IPM_Line_C0, IPM_Line_C1, IPM_Line_C2, 0]);
        end
    end
end

== stateflow chart ALL_JP360_DBW_V6_5_1103/ACC_Control/ACC_FUNCTION/Subsystem2/ACC_model/TIS1 ACC action/Subsystem1/mode change/Chart1 ==
  state a
    state OFF1
      y=0;
    state ON
      y=1;
    a -> (junction 1)
    (junction 1) -> OFF1 [order 2]
    (default) -> (junction 1)
    (junction 1) -> ON [order 1] : [acc_obj_detected==0||(acc_obj_detected==1&&v_obj>v_set)]
  (default) -> a
  data: acc_obj_detected input; v_obj input; v_set input; y output int8

== matlab function ALL_JP360_DBW_V6_5_1103/ACC_Control/ACC_FUNCTION/Subsystem2/ACC_model/TIS1 ACC action/Subsystem1/mode change/cc and close and follow/cc and close/move close/MATLAB Function ==
  data: delta_d input; y output
function y = fcn(delta_d)
    if abs(delta_d) >= 1
        y = delta_d;
    elseif delta_d < 1 && delta_d>=0
        y = single(1);
    else 
        y = single(-1);
    end
end

== matlab function ALL_JP360_DBW_V6_5_1103/ACC_Control/ACC_FUNCTION/Subsystem2/ACC_model/TIS1 ACC action/Subsystem1/mode change/cc and close and follow/cc and close/move close/MATLAB Function1 ==
  data: delta_v input; acc output; dx input; a_dem input; dec output; a_close input; cc_throttle input; cc_brake input
function [acc, dec] = fcn(delta_v, dx, a_dem, a_close, cc_throttle, cc_brake)
    if 50 >= dx
        acc = single(0);
        dec = a_close;
    else
        acc = cc_throttle;
        dec = cc_brake;
    end
end

== matlab function ALL_JP360_DBW_V6_5_1103/CIPV1/Lane Line Construction1/Embedded MATLAB Function7 ==
  data: judge output; IPM_Line_type input; IPM_Line_Existence_Probability input; IPM_Line_C0 input; line_data output; IPM_Line_C1 input; IPM_Line_C2 input; IPM_Line_C3 input; judge_cover_line_left input; judge_cover_line_right input
function [judge, line_data] = line_fun(IPM_Line_type, IPM_Line_Existence_Probability, IPM_Line_C0, IPM_Line_C1, IPM_Line_C2, IPM_Line_C3, judge_cover_line_left, judge_cover_line_right)

judge = 0;
% Judge whether it is a road edge
if IPM_Line_type == 2
    line_data = single([0, 0, 0, 0]);
else
    if IPM_Line_Existence_Probability >= 0.5 && judge_cover_line_left==0 && judge_cover_line_right==0
        line_data = single([IPM_Line_C0, IPM_Line_C1, IPM_Line_C2, IPM_Line_C3]);
        judge = 1;
    else
        line_data = single([0,0,0,0]);
        judge = 0;
    end
end
end

== matlab function ALL_JP360_DBW_V6_5_1103/CIPV1/Lane Line Construction1/Embedded MATLAB Function8 ==
  data: R input; SteerWheelAngle input; line_data output; IPM_Line_type input
function line_data = line_count_fun(R, SteerWheelAngle, IPM_Line_type)

if IPM_Line_type==2   %右车道线是道路边缘，所以无右右车道线
    line_data = single([0, 0, 0, 0]);
else
    if R>100
        line_data = single([-5.625, 0, 0, 0]);
    else
        if SteerWheelAngle < 0  %turn right
            IPM_Line_C0 = -5.625;
            IPM_Line_C1 = 0;
            IPM_Line_C2 = -(1/(R-5.625));
            line_data = single([IPM_Line_C0, IPM_Line_C1, IPM_Line_C2, 0]);
        else
            IPM_Line_C0 = -5.625;
            IPM_Line_C1 = 0;
            IPM_Line_C2 = 1/(R+5.625);
            line_data = single([IPM_Line_C0, IPM_Line_C1, IPM_Line_C2, 0]);
        end
    end
end

== matlab function ALL_JP360_DBW_V6_5_1103/CIPV1/Lane Line Construction1/Embedded MATLAB Function9 ==
  data: IPM_Line_Existence_Probability input; IPM_Line_C0 input; judge_cover_line output; IPM_Line_C1 input; IPM_Line_C2 input; IPM_Line_C3 input
function judge_cover_line = line_fun(IPM_Line_Existence_Probability, IPM_Line_C0, IPM_Line_C1, IPM_Line_C2, IPM_Line_C3)
x = 4.174;
y = 1.083;
if IPM_Line_Existence_Probability >= 0.5
    y_ = IPM_Line_C0 + IPM_Line_C1*x + IPM_Line_C2/2*x^2 + IPM_Line_C3/6*x^3;  %判断是否压线
    if y_<y   %压线
        judge_cover_line = 1;
    else
        judge_cover_line = 0;

    end
else
    judge_cover_line = 1;
end

== matlab function ALL_JP360_DBW_V6_5_1103/CIPV1/Obstacle selection/Subsystem/Subsystem/MATLAB Function ==
  data: mrr_type input; y output; ipm_id input; ipm_obj input; hasCamera input
function y = fcn(mrr_type,ipm_id,ipm_obj,hasCamera)
if hasCamera==0 ||mrr_type~=7
    y=mrr_type;
    return;
else
for i=0:19
    if(ipm_id==ipm_obj(i*16+4))
        if(ipm_obj(i*16+9)==2)
            y=single(6);
            return;
        else
            y=mrr_type;
            return;
        end
    end
end
end
y=mrr_type;

== matlab function ALL_JP360_DBW_V6_5_1103/CIPV1/Obstacle selection/Subsystem/Subsystem1/MATLAB Function ==
  data: mrr_type input; y output; ipm_id input; ipm_obj input; hasCamera input
function y = fcn(mrr_type,ipm_id,ipm_obj,hasCamera)
if hasCamera==0 ||mrr_type~=7
    y=mrr_type;
    return;
else
for i=0:19
    if(ipm_id==ipm_obj(i*16+4))
        if(ipm_obj(i*16+9)==2)
            y=single(6);
            return;
        else
            y=mrr_type;
            return;
        end
    end
end
end
y=mrr_type;

== matlab function ALL_JP360_DBW_V6_5_1103/CIPV1/Obstacle selection/Subsystem/Subsystem2/MATLAB Function ==
  data: mrr_type input; y output; ipm_id input; ipm_obj input; hasCamera input
function y = fcn(mrr_type,ipm_id,ipm_obj,hasCamera)
if hasCamera==0 ||mrr_type~=7
    y=mrr_type;
    return;
else
for i=0:19
    if(ipm_id==ipm_obj(i*16+4))
        if(ipm_obj(i*16+9)==2)
            y=single(6);
            return;
        else
            y=mrr_type;
            return;
        end
    end
end
end
y=mrr_type;

== matlab function ALL_JP360_DBW_V6_5_1103/CIPV1/Obstacle selection/Subsystem/Subsystem3/MATLAB Function ==
  data: mrr_type input; y output; ipm_id input; ipm_obj input; hasCamera input
function y = fcn(mrr_type,ipm_id,ipm_obj,hasCamera)
if hasCamera==0 ||mrr_type~=7
    y=mrr_type;
    return;
else
for i=0:19
    if(ipm_id==ipm_obj(i*16+4))
        if(ipm_obj(i*16+9)==2)
            y=single(6);
            return;
        else
            y=mrr_type;
            return;
        end
    end
end
end
y=mrr_type;

== matlab function ALL_JP360_DBW_V6_5_1103/CIPV1/Obstacle selection/Subsystem1/If Action Subsystem2/MATLAB Function ==
  data: IPM_Obj input; MRR_ObjID output; last_cipv1_MRR_ObjFusionCamID input; last_cipv1_MRR_ObjFusionSig input; last_cipv1_MRR_ObjID input; MRR_ObjDistX output; MRR_ObjDistY output; MRR_ObjRelVelX output; MRR_ObjRelVelY output; MRR_ObjType output; MRR_ObjUpdFlg output; obj_vaild output; untracktime output; MRR_ObjFusionCamID output; MRR_ObjFusionSig output; last_cipv1_MRR_ObjDistX input; last_cipv1_MRR_ObjDistY input; last_cipv1_MRR_ObjRelVelX input; last_cipv1_MRR_ObjRelVelY input; last_cipv1_MRR_ObjType input; last_cipv1_MRR_ObjUpdFlg input; last_cipv1_obj_vaild input; last_cipv1_untracktime input
function [MRR_ObjID,MRR_ObjDistX,MRR_ObjDistY,MRR_ObjRelVelX,MRR_ObjRelVelY,MRR_ObjType,MRR_ObjUpdFlg,obj_vaild,untracktime,MRR_ObjFusionCamID,MRR_ObjFusionSig]= fcn(IPM_Obj, ...
    last_cipv1_MRR_ObjFusionCamID,last_cipv1_MRR_ObjFusionSig,last_cipv1_MRR_ObjID, last_cipv1_MRR_ObjDistX, last_cipv1_MRR_ObjDistY, ...
    last_cipv1_MRR_ObjRelVelX, last_cipv1_MRR_ObjRelVelY, ...
    last_cipv1_MRR_ObjType, last_cipv1_MRR_ObjUpdFlg, last_cipv1_obj_vaild, last_cipv1_untracktime)
if last_cipv1_MRR_ObjFusionSig~=0
    for i=0:19
    if(last_cipv1_MRR_ObjFusionCamID==IPM_Obj(i*16+4))
        if(IPM_Obj(i*16+11)>90)
            MRR_ObjID=last_cipv1_MRR_ObjID;
            MRR_ObjDistX=IPM_Obj(i*16+2);
            MRR_ObjDistY=IPM_Obj(i*16+3);
            MRR_ObjRelVelX=IPM_Obj(i*16+7);
            MRR_ObjRelVelY=IPM_Obj(i*16+8);
            MRR_ObjType=last_cipv1_MRR_ObjType;
            MRR_ObjUpdFlg=last_cipv1_MRR_ObjUpdFlg;
            obj_vaild=last_cipv1_obj_vaild;
            untracktime=single(0);
            MRR_ObjFusionCamID=last_cipv1_MRR_ObjFusionCamID;
            MRR_ObjFusionSig=last_cipv1_MRR_ObjFusionSig;
            return
        end
    end

    end
end
            MRR_ObjID=last_cipv1_MRR_ObjID;
            MRR_ObjDistX=last_cipv1_MRR_ObjDistX;
            MRR_ObjDistY=last_cipv1_MRR_ObjDistY;
            MRR_ObjRelVelX=last_cipv1_MRR_ObjRelVelX;
            MRR_ObjRelVelY=last_cipv1_MRR_ObjRelVelY;
            MRR_ObjType=last_cipv1_MRR_ObjType;
            MRR_ObjUpdFlg=last_cipv1_MRR_ObjUpdFlg;
            obj_vaild=last_cipv1_obj_vaild;
            untracktime=last_cipv1_untracktime;
            MRR_ObjFusionCamID=last_cipv1_MRR_ObjFusionCamID;
            MRR_ObjFusionSig=last_cipv1_MRR_ObjFusionSig;

== matlab function ALL_JP360_DBW_V6_5_1103/CIPV1/getMrrObjFcn ==
  data: y1 output; u input; y2 output; y3 output; y4 output; y5 output; y6 output; y7 output; y8 output; y9 output; y10 output; y11 output; y12 output; y13 output; y14 output
function [y1,y2, y3,y4,y5,y6,y7,y8,y9,y10,y11,y12,y13,y14] = fcn(u)
    
y1 = reshape(single(u(1,:)),[],1);
y2 = reshape(single(u(2,:)),[],1);
y3 = reshape(single(u(3,:)),[],1);
y4 = reshape(single(u(4,:)),[],1);
y5 = reshape(single(u(5,:)),[],1);
y6 = reshape(single(u(6,:)),[],1);
y7 = reshape(single(u(7,:)),[],1);
y8 = reshape(single(u(8,:)),[],1);
y9 = reshape(single(u(9,:)),[],1);
y10 = reshape(single(u(10,:)),[],1);
y11 = reshape(single(u(11,:)),[],1);
y12 = reshape(single(u(12,:)),[],1);
y13 = reshape(single(u(13,:)),[],1);
y14 = reshape(single(u(14,:)),[],1);
end
